simulink model "SIL_Formulas"  (R2025b)
settings: Solver=VariableStepAuto  StartTime=0.0  StopTime=10.0  RelTol=1e-3
settings Model: Creator=BillL  LastModifiedBy=BillL

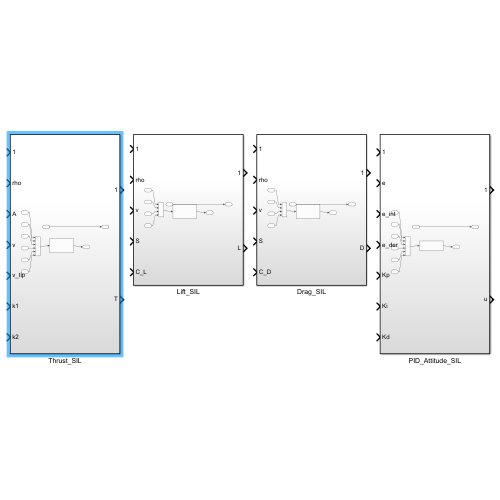
[thumbnail: Simulink's stored preview of the top-level diagram]
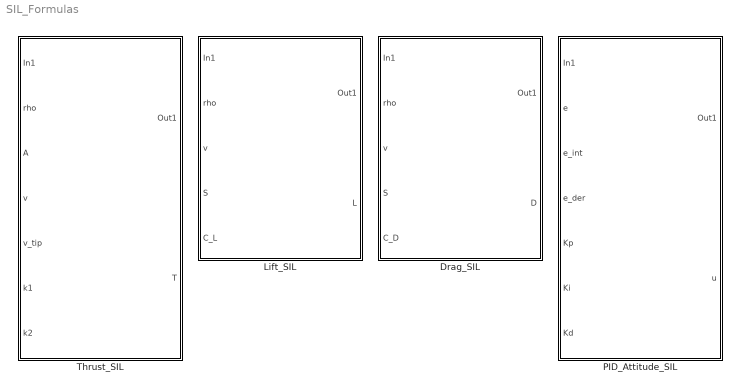
== system SIL_Formulas ==
  Drag_SIL : Subsystem
  Lift_SIL : Subsystem
  PID_Attitude_SIL : Subsystem
  Thrust_SIL : Subsystem

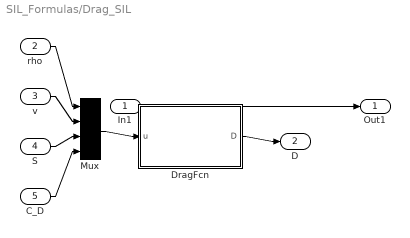
== system SIL_Formulas/Drag_SIL ==
  In1 : Inport
  rho : Inport  Port=2
  v : Inport  Port=3
  S : Inport  Port=4
  C_D : Inport  Port=5
  DragFcn : MATLAB Function  TreatAsAtomicUnit=on
  Mux : Mux
  Out1 : Outport
  D : Outport  Port=2
  wires:
  In1/1 -> Out1/1
  rho/1 -> Mux/1
  v/1 -> Mux/2
  S/1 -> Mux/3
  C_D/1 -> Mux/4
  Mux/1 -> DragFcn/1(u)
  DragFcn/1(D) -> D/1

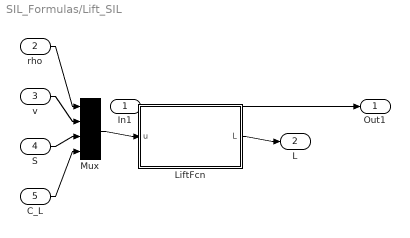
== system SIL_Formulas/Lift_SIL ==
  In1 : Inport
  rho : Inport  Port=2
  v : Inport  Port=3
  S : Inport  Port=4
  C_L : Inport  Port=5
  LiftFcn : MATLAB Function  TreatAsAtomicUnit=on
  Mux : Mux
  Out1 : Outport
  L : Outport  Port=2
  wires:
  In1/1 -> Out1/1
  rho/1 -> Mux/1
  v/1 -> Mux/2
  S/1 -> Mux/3
  C_L/1 -> Mux/4
  Mux/1 -> LiftFcn/1(u)
  LiftFcn/1(L) -> L/1

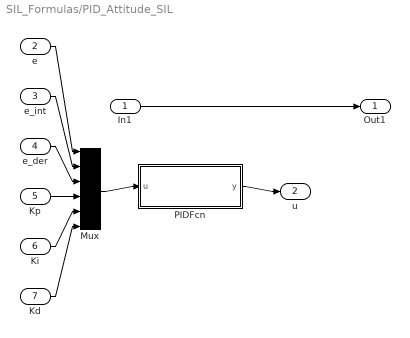
== system SIL_Formulas/PID_Attitude_SIL ==
  In1 : Inport
  e : Inport  Port=2
  e_int : Inport  Port=3
  e_der : Inport  Port=4
  Kp : Inport  Port=5
  Ki : Inport  Port=6
  Kd : Inport  Port=7
  Mux : Mux  Inputs=6
  PIDFcn : MATLAB Function  TreatAsAtomicUnit=on
  Out1 : Outport
  u : Outport  Port=2
  wires:
  In1/1 -> Out1/1
  e/1 -> Mux/1
  e_int/1 -> Mux/2
  e_der/1 -> Mux/3
  Kp/1 -> Mux/4
  Ki/1 -> Mux/5
  Kd/1 -> Mux/6
  Mux/1 -> PIDFcn/1(u)
  PIDFcn/1(y) -> u/1

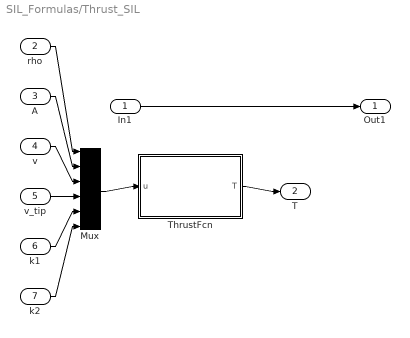
== system SIL_Formulas/Thrust_SIL ==
  In1 : Inport
  rho : Inport  Port=2
  A : Inport  Port=3
  v : Inport  Port=4
  v_tip : Inport  Port=5
  k1 : Inport  Port=6
  k2 : Inport  Port=7
  Mux : Mux  Inputs=6
  ThrustFcn : MATLAB Function  TreatAsAtomicUnit=on
  Out1 : Outport
  T : Outport  Port=2
  wires:
  In1/1 -> Out1/1
  rho/1 -> Mux/1
  A/1 -> Mux/2
  v/1 -> Mux/3
  v_tip/1 -> Mux/4
  k1/1 -> Mux/5
  k2/1 -> Mux/6
  Mux/1 -> ThrustFcn/1(u)
  ThrustFcn/1(T) -> T/1

== matlab function SIL_Formulas/Thrust_SIL/ThrustFcn ==
  data: u input; T output
function T = thrust_block(u)
rho = u(1); A = u(2); v = u(3); v_tip = u(4); k1 = u(5); k2 = u(6);
if v_tip <= 0
    C_T = 0;
else
    ratio = v / v_tip;
    C_T = k1 * ratio + k2 * ratio^2;
end
T = 0.5 * rho * A * v^2 * C_T;
end

== matlab function SIL_Formulas/Drag_SIL/DragFcn ==
  data: u input; D output
function D = drag_block(u)
D = 0.5 * u(1) * u(2)^2 * u(3) * u(4);
end

== matlab function SIL_Formulas/PID_Attitude_SIL/PIDFcn ==
  data: u input; y output
function y = pid_block(u)
y = u(4)*u(1) + u(5)*u(2) + u(6)*u(3);
end

== matlab function SIL_Formulas/Lift_SIL/LiftFcn ==
  data: u input; L output
function L = lift_block(u)
L = 0.5 * u(1) * u(2)^2 * u(3) * u(4);
end
